simulink model "chua_sim_2014"  (R2014a)
settings: Solver=ode23t  SolverMode=SingleTasking  StartTime=0.0  StopTime=Tfin  RelTol=1e-3
values from neighbouring files (symbols this model uses):
  x0 = randn(3,1)*0.2    [main_chua.m]
  xp0 = x0+[0.01;0;0]    [main_chua.m]
undefined symbols (not defined in the file or in its folder): fg_chua
settings Model: CovMetricSettings=dwe  CovHtmlReporting=off  covSaveCumulativeToWorkspaceVar=off  CovSaveSingleToWorkspaceVar=off  CovExternalEMLEnable=on  CovSFcnEnable=on  Creator=carlonovara  LastModifiedBy=carlonovara
settings DataIOCC: LimitDataPoints=off  SaveFormat=StructureWithTime
settings DebuggingCC: MergeDetectMultiDrivingBlocksExec=error  SolverPrmCheckMsg=none  FrameProcessingCompatibilityMsg=error  SFUnexpectedBacktrackingDiag=error  SFNoUnconditionalDefaultTransitionDiag=error
settings HardwareCC: ProdBitPerPointer=64  ProdLargestAtomicFloat=Float  ProdIntDivRoundTo=Zero  ProdEndianess=LittleEndian  ProdHWDeviceType=Specified
settings ModelReferenceCC: PropagateSignalLabelsOutOfModel=on
settings GRTTargetCC: TargetLangStandard=C99 (ISO)  GeneratePreprocessorConditionals=Use local settings

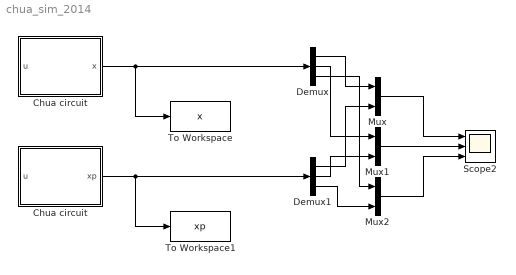
== system chua_sim_2014 ==
  Chua circuit : Subsystem
  "Chua circuit " : Subsystem
  Demux : Demux  Outputs=3
  Demux1 : Demux  Outputs=3
  Mux : Mux  Inputs=2
  Mux1 : Mux  Inputs=2
  Mux2 : Mux  Inputs=2
  Scope2 : Scope  NumInputPorts=3
      settings: TimeRange=auto  MaxDataPoints=5000  SaveToWorkspace=off  SaveName=ScopeData  YMin=-1.04734~-0.1567~-0.20912  YMax=0.11849~0.18726~1.44915  SampleTime=-1
  To Workspace : ToWorkspace  VariableName=x  SampleTime=-1
  To Workspace1 : ToWorkspace  VariableName=xp  SampleTime=-1
  wires:
  Chua circuit/1(x) -> To Workspace/1, Demux/1
  "Chua circuit "/1(xp) -> To Workspace1/1, Demux1/1
  Mux/1 -> Scope2/1
  Mux1/1 -> Scope2/2
  Mux2/1 -> Scope2/3
  Demux/1 -> Mux/1
  Demux1/1 -> Mux/2
  Demux/2 -> Mux1/1
  Demux1/2 -> Mux1/2
  Demux/3 -> Mux2/1
  Demux1/3 -> Mux2/2

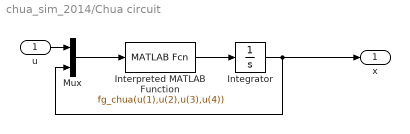
== system chua_sim_2014/Chua circuit ==
  u : Inport
  Integrator : Integrator  InitialCondition=x0
  Interpreted MATLAB Function : MATLABFcn  MATLABFcn=fg_chua(u(1),u(2),u(3),u(4))  OutputDimensions=3
  Mux : Mux  Inputs=2
  x : Outport
  wires:
  u/1 -> Mux/1
  Interpreted MATLAB Function/1 -> Integrator/1
  Integrator/1 -> Mux/2, x/1
  Mux/1 -> Interpreted MATLAB Function/1

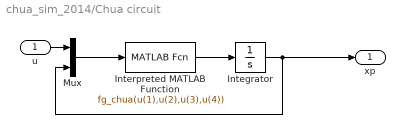
== system chua_sim_2014/Chua circuit  ==
  u : Inport
  Integrator : Integrator  InitialCondition=xp0
  Interpreted MATLAB Function : MATLABFcn  MATLABFcn=fg_chua(u(1),u(2),u(3),u(4))  OutputDimensions=3
  Mux : Mux  Inputs=2
  xp : Outport
  wires:
  Mux/1 -> Interpreted MATLAB Function/1
  Integrator/1 -> Mux/2, xp/1
  Interpreted MATLAB Function/1 -> Integrator/1
  u/1 -> Mux/1
